simulink library "roller485lib"  (R2023a)
settings: Solver=VariableStepAuto  StartTime=0.0  StopTime=10.0  RelTol=1e-3
libraries: arduinolib x173, simulink x66
(part 2 of 6)

== system roller485lib/I2C Write ==
  note: position mode
  note: current mode
  note: speed mode
  absolute angle command [deg] : Subsystem  mask(absolute angle command [deg]){I2CAddress=0x64, I2CModule=0, position_P=15, position_I=0.000003, position_D=400, set_time1=0, set_time2=0}
      mask prompts: I2CAddress "I2C Address"; I2CModule "I2C Module"; position_P "P"; position_I "I"; position_D "D"; set_time1 "Set Time1"; set_time2 "Set Time2"
      mask help:
      | position mode
      | If t ≤ set_time1, then position mode is set.
      | ---------------------------------
      | default value (PID gain of position controller)
      |  P: 15
      |  I: 0.000003
      |  D: 400
      | If t ≤ set_time2, then PID gain can be set.
      mask TypeOptions I2CModule:
      | Enabled Subsystem
      | (PID setting)/I2C Write
      | (0xA0)/I2CModule | Enabled Subsystem
      | (PID setting)/I2C Write
      | (0xA4)/I2CModule | Enabled Subsystem
      | (PID setting)/I2C Write
      | (0xA8)/I2CModule | Enabled Subsystem
      | (mode setting)/I2C Write
      | (0x01)/I2CModule | I2C Write
      | (0x80)/I2CModule
      mask DialogControl ParameterGroupVar Prompt: パラメーター
      mask Display:
      | image('roller485.png', [55,10,75,56]);
      | 
      | color('blue');
      | text(5, 62, 'absolute position control');
      | text(17, 22, '# mode setting');
      | text(17, 10, '# PID gain setting');
      | color('black');
      | 
      | color('red');
      | addr = get_param(gcb, 'I2CAddress');
      | text(10, 50, ['I2C: ' addr]);
      | 
      | color('red');
      | module = get_param(gcb, 'I2CModule');
      | text(60, 50, ['<I2C' module '>']);
  absolute angle command [deg] and max current [mA] : Subsystem  mask(absolute angle command [deg]){I2CAddress=0x64, I2CModule=0, position_P=15, position_I=0.000003, position_D=400, max_current=1000, set_time1=0, set_time2=0, set_time3=0}
      mask prompts: I2CAddress "I2C Address"; I2CModule "I2C Module"; position_P "P"; position_I "I"; position_D "D"; max_current "Imax [mA]"; set_time1 "Set Time1"; set_time2 "Set Time2"; set_time3 "Set Time3"
      mask help:
      | position mode
      | If t ≤ set_time1, then position mode is set.
      | ---------------------------------
      | default value (PID gain of position controller)
      |  P: 15
      |  I: 0.000003
      |  D: 400
      | If t ≤ set_time2, then PID gain can be set.
      | ---------------------------------
      | default value (Imax: max current)
      |  Imax: 1000 mA
      |   ---> Imax can be set up to a maximum of 1200mA.
      | If t ≤ set_time3, then Imax can be set.
      mask TypeOptions I2CModule:
      | Enabled Subsystem
      | (PID setting)/I2C Write
      | (0xA0)/I2CModule | Enabled Subsystem
      | (PID setting)/I2C Write
      | (0xA4)/I2CModule | Enabled Subsystem
      | (PID setting)/I2C Write
      | (0xA8)/I2CModule | Enabled Subsystem
      | (max current setting)/I2C Write
      | (0x50)/I2CModule | Enabled Subsystem
      | (mode setting)/I2C Write
      | (0x01)/I2CModule | I2C Write
      | (0x80)/I2CModule
      mask DialogControl ParameterGroupVar Prompt: パラメーター
      mask Display:
      | image('roller485.png', [55,10,75,56]);
      | 
      | color('blue');
      | text(5, 62, 'absolute position control');
      | text(17, 22, '# mode setting');
      | text(17, 10, '# PID gain & Imax setting');
      | 
      | color('red');
      | addr = get_param(gcb, 'I2CAddress');
      | text(10, 50, ['I2C: ' addr]);
      | 
      | color('red');
      | module = get_param(gcb, 'I2CModule');
      | text(60, 50, ['<I2C' module '>']);
  absolute angle command [rad] : Subsystem  mask(absolute angle command [rad]){I2CAddress=0x64, I2CModule=0, position_P=15, position_I=0.000003, position_D=400, set_time1=0, set_time2=0}
      mask prompts: I2CAddress "I2C Address"; I2CModule "I2C Module"; position_P "P"; position_I "I"; position_D "D"; set_time1 "Set Time1"; set_time2 "Set Time2"
      mask help:
      | position mode
      | If t ≤ set_time1, then position mode is set.
      | ---------------------------------
      | default value (PID gain of position controller)
      |  P: 15
      |  I: 0.000003
      |  D: 400
      | If t ≤ set_time2, then PID gain can be set.
      mask TypeOptions I2CModule:
      | Enabled Subsystem
      | (PID setting)/I2C Write
      | (0xA0)/I2CModule | Enabled Subsystem
      | (PID setting)/I2C Write
      | (0xA4)/I2CModule | Enabled Subsystem
      | (PID setting)/I2C Write
      | (0xA8)/I2CModule | Enabled Subsystem
      | (mode setting)/I2C Write
      | (0x01)/I2CModule | I2C Write
      | (0x80)/I2CModule
      mask DialogControl ParameterGroupVar Prompt: パラメーター
      mask Display:
      | image('roller485.png', [55,10,75,56]);
      | 
      | color('blue');
      | text(5, 62, 'absolute position control');
      | text(17, 22, '# mode setting');
      | text(17, 10, '# PID gain setting');
      | 
      | color('red');
      | addr = get_param(gcb, 'I2CAddress');
      | text(10, 50, ['I2C: ' addr]);
      | 
      | color('red');
      | module = get_param(gcb, 'I2CModule');
      | text(60, 50, ['<I2C' module '>']);
  absolute angle command [rad] and max current [mA] : Subsystem  mask(absolute angle command [rad]){I2CAddress=0x64, I2CModule=0, position_P=15, position_I=0.000003, position_D=400, max_current=1000, set_time1=0, set_time2=0, set_time3=0}
      mask prompts: I2CAddress "I2C Address"; I2CModule "I2C module:"; position_P "P"; position_I "I"; position_D "D"; max_current "Imax [mA]"; set_time1 "Set Time1"; set_time2 "Set Time2"; set_time3 "Set Time3"
      mask help:
      | position mode
      | If t ≤ set_time1, then position mode is set.
      | ---------------------------------
      | default value (PID gain of position controller)
      |  P: 15
      |  I: 0.000003
      |  D: 400
      | If t ≤ set_time2, then PID gain can be set.
      | ---------------------------------
      | default value (Imax: max current)
      |  Imax: 1000 mA
      |   ---> Imax can be set up to a maximum of 1200mA.
      | If t ≤ set_time3, then Imax can be set.
      mask TypeOptions I2CModule:
      | Enabled Subsystem
      | (PID setting)/I2C Write
      | (0xA0)/I2CModule | Enabled Subsystem
      | (PID setting)/I2C Write
      | (0xA4)/I2CModule | Enabled Subsystem
      | (PID setting)/I2C Write
      | (0xA8)/I2CModule | Enabled Subsystem
      | (max current setting)/I2C Write
      | (0x50)/I2CModule | Enabled Subsystem
      | (mode setting)/I2C Write
      | (0x01)/I2CModule | I2C Write
      | (0x80)/I2CModule
      mask DialogControl ParameterGroupVar Prompt: パラメーター
      mask Display:
      | image('roller485.png', [55,10,75,56]);
      | 
      | color('blue');
      | text(5, 62, 'absolute position control');
      | text(17, 22, '# mode setting');
      | text(17, 10, '# PID gain & Imax setting');
      | 
      | color('red');
      | addr = get_param(gcb, 'I2CAddress');
      | text(10, 50, ['I2C: ' addr]);
      | 
      | color('red');
      | module = get_param(gcb, 'I2CModule');
      | text(60, 50, ['<I2C' module '>']);
  angular velocity command [rad/s] : Subsystem  mask(angular velocity command [rad/s]){I2CAddress=0x64, I2CModule=0, speed_P=15, speed_I=0.0001, speed_D=400, set_time1=0, set_time2=0}
      mask prompts: I2CAddress "I2C Address"; I2CModule "I2C Module"; speed_P "P"; speed_I "I"; speed_D "D"; set_time1 "Set Time1"; set_time2 "Set Time2"
      mask help:
      | speed mode
      | If t ≤ set_time1, then speed mode is set.
      | ---------------------------------
      | default value (PID gain of speed controller)
      |      P: 15,  I: 0.0001,  D: 400
      | recommended value (PID gain of speed controller)
      |      P: 2,  I: 0,  D: 850
      | If t ≤ set_time2, then PID gain can be set.
      mask TypeOptions I2CModule:
      | Enabled Subsystem
      | (PID setting)/I2C Write
      | (0x70)/I2CModule | Enabled Subsystem
      | (PID setting)/I2C Write
      | (0x74)/I2CModule | Enabled Subsystem
      | (PID setting)/I2C Write
      | (0x78)/I2CModule | Enabled Subsystem
      | (mode setting)/I2C Write
      | (0x01)/I2CModule | I2C Write
      | (0x40)/I2CModule
      mask DialogControl ParameterGroupVar Prompt: パラメーター
      mask Display:
      | image('roller485.png', [55,10,75,56]);
      | 
      | color('green');
      | text(5, 62, 'speed control');
      | text(17, 22, '# mode setting');
      | text(17, 10, '# PID gain setting');
      | 
      | color('red');
      | addr = get_param(gcb, 'I2CAddress');
      | text(10, 50, ['I2C: ' addr]);
      | 
      | color('red');
      | module = get_param(gcb, 'I2CModule');
      | text(60, 50, ['<I2C' module '>']);
  angular velocity command [rad/s] and max current [mA] : Subsystem  mask(angular velocity command [rad/s]){I2CAddress=0x64, I2CModule=0, speed_P=15, speed_I=0.0001, speed_D=400, max_current=1000, set_time1=0, set_time2=0, set_time3=0}
      mask prompts: I2CAddress "I2C Address"; I2CModule "I2C Module"; speed_P "P"; speed_I "I"; speed_D "D"; max_current "Imax [mA]"; set_time1 "Set Time1"; set_time2 "Set Time2"; set_time3 "Set Time3"
      mask help:
      | speed mode
      | If t ≤ set_time1, then speed mode is set.
      | ---------------------------------
      | default value (PID gain of speed controller)
      |      P: 15,  I: 0.0001,  D: 400
      | recommended value (PID gain of speed controller)
      |      P: 2,  I: 0,  D: 850
      | If t ≤ set_time2, then PID gain and Imax can be set.
      | ---------------------------------
      | default value (Imax: max current)
      |  Imax: 1000 mA
      |  ---> Imax can be set up to a maximum of 1200mA.
      | If t ≤ set_time3, then Imax is set.
      mask TypeOptions I2CModule:
      | Enabled Subsystem
      | (PID setting)/I2C Write
      | (0x70)/I2CModule | Enabled Subsystem
      | (PID setting)/I2C Write
      | (0x74)/I2CModule | Enabled Subsystem
      | (PID setting)/I2C Write
      | (0x78)/I2CModule | Enabled Subsystem
      | (max current setting)/I2C Write
      | (0x50)/I2CModule | Enabled Subsystem
      | (mode setting)/I2C Write
      | (0x01)/I2CModule | I2C Write
      | (0x40)/I2CModule
      mask DialogControl ParameterGroupVar Prompt: パラメーター
      mask Display:
      | image('roller485.png', [55,10,75,56]);
      | 
      | color('green');
      | text(5, 62, 'speed control');
      | text(17, 22, '# mode setting');
      | text(17, 10, '# PID gain & Imax setting');
      | 
      | color('red');
      | addr = get_param(gcb, 'I2CAddress');
      | text(10, 50, ['I2C: ' addr]);
      | 
      | color('red');
      | module = get_param(gcb, 'I2CModule');
      | text(60, 50, ['<I2C' module '>']);
  angular velocity command [rpm] : Subsystem  mask(angular velocity command [rad/s]){I2CAddress=0x64, I2CModule=0, speed_P=15, speed_I=0.0001, speed_D=400, set_time1=0, set_time2=0}
      mask prompts: I2CAddress "I2C Address"; I2CModule "I2C Module"; speed_P "P"; speed_I "I"; speed_D "D"; set_time1 "Set Time1"; set_time2 "Set Time2"
      mask help:
      | speed mode
      | If t ≤ set_time1, then speed mode is set.
      | ---------------------------------
      | default value (PID gain of speed controller)
      |      P: 15,  I: 0.0001,  D: 400
      | recommended value (PID gain of speed controller)
      |      P: 2,  I: 0,  D: 850
      | If t ≤ set_time2, then PID gain can be set.
      mask TypeOptions I2CModule:
      | Enabled Subsystem
      | (PID setting)/I2C Write
      | (0x70)/I2CModule | Enabled Subsystem
      | (PID setting)/I2C Write
      | (0x74)/I2CModule | Enabled Subsystem
      | (PID setting)/I2C Write
      | (0x78)/I2CModule | Enabled Subsystem
      | (mode setting)/I2C Write
      | (0x01)/I2CModule | I2C Write
      | (0x40)/I2CModule
      mask DialogControl ParameterGroupVar Prompt: パラメーター
      mask Display:
      | image('roller485.png', [55,10,75,56]);
      | 
      | color('green');
      | text(5, 62, 'speed control');
      | text(17, 22, '# mode setting');
      | text(17, 10, '# PID gain setting');
      | 
      | color('red');
      | addr = get_param(gcb, 'I2CAddress');
      | text(10, 50, ['I2C: ' addr]);
      | 
      | color('red');
      | module = get_param(gcb, 'I2CModule');
      | text(60, 50, ['<I2C' module '>']);
  angular velocity command [rpm] and max current [mA] : Subsystem  mask(angular velocity command [rpm]){I2CAddress=0x64, I2CModule=0, speed_P=15, speed_I=0.0001, speed_D=400, max_current=1000, set_time1=0, set_time2=0, set_time3=0}
      mask prompts: I2CAddress "I2C Address"; I2CModule "I2C Module"; speed_P "P"; speed_I "I"; speed_D "D"; max_current "Imax [mA]"; set_time1 "Set Time1"; set_time2 "Set Time2"; set_time3 "Set Time3"
      mask help:
      | speed mode
      | If t ≤ set_time1, then speed mode is set.
      | ---------------------------------
      | default value (PID gain of speed controller)
      |      P: 15,  I: 0.0001,  D: 400
      | recommended value (PID gain of speed controller)
      |      P: 2,  I: 0,  D: 850
      | If t ≤ set_time2, then PID gain and Imax can be set.
      | ---------------------------------
      | default value (Imax: max current)
      |  Imax: 1000 mA
      |  ---> Imax can be set up to a maximum of 1200mA.
      | If t ≤ set_time3, then Imax is set.
      mask TypeOptions I2CModule:
      | Enabled Subsystem
      | (PID setting)/I2C Write
      | (0x70)/I2CModule | Enabled Subsystem
      | (PID setting)/I2C Write
      | (0x74)/I2CModule | Enabled Subsystem
      | (PID setting)/I2C Write
      | (0x78)/I2CModule | Enabled Subsystem
      | (max current setting)/I2C Write
      | (0x50)/I2CModule | Enabled Subsystem
      | (mode setting)/I2C Write
      | (0x01)/I2CModule | I2C Write
      | (0x40)/I2CModule
      mask DialogControl ParameterGroupVar Prompt: パラメーター
      mask Display:
      | image('roller485.png', [55,10,75,56]);
      | color('green');
      | text(5, 62, 'speed control');
      | 
      | text(17, 22, '# mode setting');
      | text(17, 10, '# PID gain & Imax setting');
      | 
      | color('red');
      | addr = get_param(gcb, 'I2CAddress');
      | text(10, 50, ['I2C: ' addr]);
      | 
      | color('red');
      | module = get_param(gcb, 'I2CModule');
      | text(60, 50, ['<I2C' module '>']);
  current command [A] : Subsystem  mask(current command [A]){I2CAddress=0x64, I2CModule=0, set_time=0}
      mask prompts: I2CAddress "I2C Address"; I2CModule "I2C Module"; set_time "Set Time"
      mask help:
      | current mode
      | If t ≤ set_time, then current mode is set.
      | ---------------------------------
      | PID gain of current controller
      |  P: 0.002
      |  I: 0.00005
      |  D: 0
      | Changing the PID gains is not permitted.
      mask TypeOptions I2CModule:
      | Enabled Subsystem
      | (mode setting)/I2C Write
      | (0x01)/I2CModule | I2C Write
      | (0xB0)/I2CModule
      mask DialogControl ParameterGroupVar Prompt: パラメーター
      mask Display:
      | image('roller485.png', [55,10,75,56]);
      | 
      | color('orange');
      | text(5, 62, 'current control');
      | text(17, 22, '# mode setting');
      | 
      | color('red');
      | addr = get_param(gcb, 'I2CAddress');
      | text(10, 50, ['I2C: ' addr]);
      | 
      | color('red');
      | module = get_param(gcb, 'I2CModule');
      | text(60, 50, ['<I2C' module '>']);
  current command [mA] : Subsystem  mask(current command [A]){I2CAddress=0x64, I2CModule=0, set_time=0}
      mask prompts: I2CAddress "I2C Address"; I2CModule "I2C Module"; set_time "Set Time"
      mask help:
      | current mode
      | If t ≤ set_time, then current mode is set.
      | ---------------------------------
      | PID gain of current controller
      |  P: 0.002
      |  I: 0.00005
      |  D: 0
      | Changing the PID gains is not permitted.
      mask TypeOptions I2CModule:
      | Enabled Subsystem
      | (mode setting)/I2C Write
      | (0x01)/I2CModule | I2C Write
      | (0xB0)/I2CModule
      mask DialogControl ParameterGroupVar Prompt: パラメーター
      mask Display:
      | image('roller485.png', [55,10,75,56]);
      | 
      | color('orange');
      | text(5, 62, 'current control');
      | text(17, 22, '# mode setting');
      | 
      | color('red');
      | addr = get_param(gcb, 'I2CAddress');
      | text(10, 50, ['I2C: ' addr]);
      | 
      | color('red');
      | module = get_param(gcb, 'I2CModule');
      | text(60, 50, ['<I2C' module '>']);
  relative angle command [deg] : Subsystem  mask(relative angle command [deg]){I2CAddress=0x64, I2CModule=0, sample_time=-1, position_P=15, position_I=0.000003, position_D=400, set_time1=0, set_time2=0}
      mask prompts: I2CAddress "I2C Address"; I2CModule "I2C Module"; sample_time "Sample Time (-1 for inherited)"; position_P "P"; position_I "I"; position_D "D"; set_time1 "Set Time1"; set_time2 "Set Time2"
      mask help:
      | position mode
      | If t ≤ set_time1, then position mode and initial angle are set.
      | ---------------------------------
      | default value (PID gain of position controller)
      |  P: 15
      |  I: 0.000003
      |  D: 400
      | If t ≤ set_time2, then PID gain can be set.
      mask TypeOptions I2CModule:
      | Enabled Subsystem
      | (PID setting)/I2C Write
      | (0xA0)/I2CModule | Enabled Subsystem
      | (PID setting)/I2C Write
      | (0xA4)/I2CModule | Enabled Subsystem
      | (PID setting)/I2C Write
      | (0xA8)/I2CModule | Enabled Subsystem
      | (initialization angle)/I2C Read
      | (0x90)/I2CModule | Enabled Subsystem
      | (mode setting)/I2C Write
      | (0x01)/I2CModule | I2C Write
      | (0x80)/I2CModule
      mask DialogControl ParameterGroupVar Prompt: パラメーター
      mask Display:
      | image('roller485.png', [55,10,75,56]);
      | 
      | color('blue');
      | text(5, 62, 'relative position control');
      | text(17, 22, '# mode setting');
      | text(17, 10, '# PID gain setting');
      | 
      | color('red');
      | addr = get_param(gcb, 'I2CAddress');
      | text(10, 50, ['I2C: ' addr]);
      | 
      | color('red');
      | module = get_param(gcb, 'I2CModule');
      | text(60, 50, ['<I2C' module '>']);
  relative angle command [deg] and max current [mA] : Subsystem  mask(relative angle command [rad]){I2CAddress=0x64, I2CModule=0, sample_time=-1, position_P=15, position_I=0.000003, position_D=400, max_current=1000, set_time1=0, set_time2=0, set_time3=0}
      mask prompts: I2CAddress "I2C Address"; I2CModule "I2C module:"; sample_time "Sample Time (-1 for inherited)"; position_P "P"; position_I "I"; position_D "D"; max_current "Imax [mA]"; set_time1 "Set Time1"; set_time2 "Set Time2"; set_time3 "Set Time3"
      mask help:
      | position mode
      | If t ≤ set_time1, then position mode and initial angle are set.
      | ---------------------------------
      | default value (PID gain of position controller)
      |  P: 15
      |  I: 0.000003
      |  D: 400
      | If t ≤ set_time2, then PID gain can be set.
      | ---------------------------------
      | default value (Imax: max current)
      |  Imax: 1000 mA
      |   ---> Imax can be set up to a maximum of 1200mA.
      | If t ≤ set_time3, then Imax can be set.
      mask TypeOptions I2CModule:
      | Enabled Subsystem
      | (PID setting)/I2C Write
      | (0xA0)/I2CModule | Enabled Subsystem
      | (PID setting)/I2C Write
      | (0xA4)/I2CModule | Enabled Subsystem
      | (PID setting)/I2C Write
      | (0xA8)/I2CModule | Enabled Subsystem
      | (initialization angle)/I2C Read
      | (0x90)/I2CModule | Enabled Subsystem
      | (max current setting)/I2C Write
      | (0x50)/I2CModule | Enabled Subsystem
      | (mode setting)/I2C Write
      | (0x01)/I2CModule | I2C Write
      | (0x80)/I2CModule
      mask DialogControl ParameterGroupVar Prompt: パラメーター
      mask Display:
      | image('roller485.png', [55,10,75,56]);
      | 
      | color('blue');
      | text(5, 62, 'relative position control');
      | text(17, 22, '# mode setting');
      | text(17, 10, '# PID gain & Imax setting');
      | 
      | color('red');
      | addr = get_param(gcb, 'I2CAddress');
      | text(10, 50, ['I2C: ' addr]);
      | 
      | color('red');
      | module = get_param(gcb, 'I2CModule');
      | text(60, 50, ['<I2C' module '>']);
  relative angle command [rad] : Subsystem  mask(relative angle command [rad]){I2CAddress=0x64, I2CModule=0, sample_time=-1, position_P=15, position_I=0.000003, position_D=400, set_time1=0, set_time2=0}
      mask prompts: I2CAddress "I2C Address"; I2CModule "I2C Module"; sample_time "Sample Time (-1 for inherited)"; position_P "P"; position_I "I"; position_D "D"; set_time1 "Set Time1"; set_time2 "Set Time2"
      mask help:
      | position mode
      | If t ≤ set_time1, then position mode and initial angle are set.
      | ---------------------------------
      | default value (PID gain of position controller)
      |  P: 15
      |  I: 0.000003
      |  D: 400
      | If t ≤ set_time2, then PID gain can be set.
      mask TypeOptions I2CModule:
      | Enabled Subsystem
      | (PID setting)/I2C Write
      | (0xA0)/I2CModule | Enabled Subsystem
      | (PID setting)/I2C Write
      | (0xA4)/I2CModule | Enabled Subsystem
      | (PID setting)/I2C Write
      | (0xA8)/I2CModule | Enabled Subsystem
      | (initialization angle)/I2C Read
      | (0x90)/I2CModule | Enabled Subsystem
      | (mode setting)/I2C Write
      | (0x01)/I2CModule | I2C Write
      | (0x80)/I2CModule
      mask DialogControl ParameterGroupVar Prompt: パラメーター
      mask Display:
      | image('roller485.png', [55,10,75,56]);
      | 
      | color('blue');
      | text(5, 62, 'relative position control');
      | text(17, 22, '# mode setting');
      | text(17, 10, '# PID gain setting');
      | 
      | color('red');
      | addr = get_param(gcb, 'I2CAddress');
      | text(10, 50, ['I2C: ' addr]);
      | 
      | color('red');
      | module = get_param(gcb, 'I2CModule');
      | text(60, 50, ['<I2C' module '>']);
  relative angle command [rad] and max current [mA] : Subsystem  mask(relative angle command [rad]){I2CAddress=0x64, I2CModule=0, sample_time=-1, position_P=15, position_I=0.000003, position_D=400, max_current=1000, set_time1=0, set_time2=0, set_time3=0}
      mask prompts: I2CAddress "I2C Address"; I2CModule "I2C Module"; sample_time "Sample Time (-1 for inherited)"; position_P "P"; position_I "I"; position_D "D"; max_current "Imax [mA]"; set_time1 "Set Time1"; set_time2 "Set Time2"; set_time3 "Set Time3"
      mask help:
      | position mode
      | If t ≤ set_time1, then position mode and initial angle are set.
      | ---------------------------------
      | default value (PID gain of position controller)
      |  P: 15
      |  I: 0.000003
      |  D: 400
      | If t ≤ set_time2, then PID gain can be set.
      | ---------------------------------
      | default value (Imax: max current)
      |  Imax: 1000 mA
      |   ---> Imax can be set up to a maximum of 1200mA.
      | If t ≤ set_time3, then Imax can be set.
      mask TypeOptions I2CModule:
      | Enabled Subsystem
      | (PID setting)/I2C Write
      | (0xA0)/I2CModule | Enabled Subsystem
      | (PID setting)/I2C Write
      | (0xA4)/I2CModule | Enabled Subsystem
      | (PID setting)/I2C Write
      | (0xA8)/I2CModule | Enabled Subsystem
      | (initialization angle)/I2C Read
      | (0x90)/I2CModule | Enabled Subsystem
      | (max current setting)/I2C Write
      | (0x50)/I2CModule | Enabled Subsystem
      | (mode setting)/I2C Write
      | (0x01)/I2CModule | I2C Write
      | (0x80)/I2CModule
      mask DialogControl ParameterGroupVar Prompt: パラメーター
      mask Display:
      | image('roller485.png', [55,10,75,56]);
      | 
      | color('blue');
      | text(5, 62, 'relative position control');
      | text(17, 22, '# mode setting');
      | text(17, 10, '# PID gain & Imax setting');
      | 
      | color('red');
      | addr = get_param(gcb, 'I2CAddress');
      | text(10, 50, ['I2C: ' addr]);
      | 
      | color('red');
      | module = get_param(gcb, 'I2CModule');
      | text(60, 50, ['<I2C' module '>']);

== system roller485lib/I2C Write (using MATLAB Function) ==
  note: speed mode
  note: current mode
  note: position mode
  absolute angle command [deg] (using MATLAB Function) : Subsystem  mask(absolute angle command [deg]){I2CAddress=0x64, I2CModule=0, position_P=15, position_I=0.000003, position_D=400, set_time1=0, set_time2=0}
      mask prompts: I2CAddress "I2C Address"; I2CModule "I2C Module"; position_P "P"; position_I "I"; position_D "D"; set_time1 "Set Time1"; set_time2 "Set Time2"
      mask help:
      | position mode
      | If t ≤ set_time1, then position mode is set.
      | ---------------------------------
      | default value (PID gain of position controller)
      |  P: 15
      |  I: 0.000003
      |  D: 400
      | If t ≤ set_time2, then PID gain can be set.
      mask TypeOptions I2CModule:
      | Enabled Subsystem
      | (PID setting)/I2C Write
      | (0xA0)/I2CModule | Enabled Subsystem
      | (PID setting)/I2C Write
      | (0xA4)/I2CModule | Enabled Subsystem
      | (PID setting)/I2C Write
      | (0xA8)/I2CModule | Enabled Subsystem
      | (mode setting)/I2C Write
      | (0x01)/I2CModule | I2C Write
      | (0x80)/I2CModule
      mask DialogControl ParameterGroupVar Prompt: パラメーター
      mask Display:
      | image('roller485_matlab_fcn2.png', [55,10,75,56]);
      | 
      | color('blue');
      | text(5, 62, 'absolute position control');
      | text(17, 22, '# mode setting');
      | text(17, 10, '# PID gain setting');
      | 
      | color('red');
      | addr = get_param(gcb, 'I2CAddress');
      | text(10, 50, ['I2C: ' addr]);
      | 
      | color('red');
      | module = get_param(gcb, 'I2CModule');
      | text(60, 50, ['<I2C' module '>']);
  absolute angle command [rad] (using MATLAB Function) : Subsystem  mask(absolute angle command [rad]){I2CAddress=0x64, I2CModule=0, position_P=15, position_I=0.000003, position_D=400, set_time1=0, set_time2=0}
      mask prompts: I2CAddress "I2C Address"; I2CModule "I2C Module"; position_P "P"; position_I "I"; position_D "D"; set_time1 "Set Time1"; set_time2 "Set Time2"
      mask help:
      | position mode
      | If t ≤ set_time1, then position mode is set.
      | ---------------------------------
      | default value (PID gain of position controller)
      |  P: 15
      |  I: 0.000003
      |  D: 400
      | If t ≤ set_time2, then PID gain can be set.
      mask TypeOptions I2CModule:
      | Enabled Subsystem
      | (PID setting)/I2C Write
      | (0xA0)/I2CModule | Enabled Subsystem
      | (PID setting)/I2C Write
      | (0xA4)/I2CModule | Enabled Subsystem
      | (PID setting)/I2C Write
      | (0xA8)/I2CModule | Enabled Subsystem
      | (mode setting)/I2C Write
      | (0x01)/I2CModule | I2C Write
      | (0x80)/I2CModule
      mask DialogControl ParameterGroupVar Prompt: パラメーター
      mask Display:
      | image('roller485_matlab_fcn2.png', [55,10,75,56]);
      | 
      | color('blue');
      | text(5, 62, 'absolute position control');
      | text(17, 22, '# mode setting');
      | text(17, 10, '# PID gain setting');
      | 
      | color('red');
      | addr = get_param(gcb, 'I2CAddress');
      | text(10, 50, ['I2C: ' addr]);
      | 
      | color('red');
      | module = get_param(gcb, 'I2CModule');
      | text(60, 50, ['<I2C' module '>']);
  angular velocity command [rad/s] (using MATLAB Function) : Subsystem  mask(angular velocity command [rad/s]){I2CAddress=0x64, I2CModule=0, speed_P=15, speed_I=0.0001, speed_D=400, set_time1=0, set_time2=0}
      mask prompts: I2CAddress "I2C Address"; I2CModule "I2C Module"; speed_P "P"; speed_I "I"; speed_D "D"; set_time1 "Set Time1"; set_time2 "Set Time2"
      mask help:
      | speed mode
      | If t ≤ set_time1, then speed mode is set.
      | ---------------------------------
      | default value (PID gain of speed controller)
      |      P: 15,  I: 0.0001,  D: 400
      | recommended value (PID gain of speed controller)
      |      P: 2,  I: 0,  D: 850
      | If t ≤ set_time2, then PID gain can be set.
      mask TypeOptions I2CModule:
      | Enabled Subsystem
      | (PID setting)/I2C Write
      | (0x70)/I2CModule | Enabled Subsystem
      | (PID setting)/I2C Write
      | (0x74)/I2CModule | Enabled Subsystem
      | (PID setting)/I2C Write
      | (0x78)/I2CModule | Enabled Subsystem
      | (mode setting)/I2C Write
      | (0x01)/I2CModule | I2C Write
      | (0x40)/I2CModule
      mask DialogControl ParameterGroupVar Prompt: パラメーター
      mask Display:
      | image('roller485_matlab_fcn2.png', [55,10,75,56]);
      | 
      | color('green');
      | text(5, 62, 'speed control');
      | text(17, 22, '# mode setting');
      | text(17, 10, '# PID gain setting');
      | 
      | color('red');
      | addr = get_param(gcb, 'I2CAddress');
      | text(10, 50, ['I2C: ' addr]);
      | 
      | color('red');
      | module = get_param(gcb, 'I2CModule');
      | text(60, 50, ['<I2C' module '>']);
  angular velocity command [rpm] (using MATLAB Function) : Subsystem  mask(angular velocity command [rpm]){I2CAddress=0x64, I2CModule=0, speed_P=15, speed_I=0.0001, speed_D=400, set_time1=0, set_time2=0}
      mask prompts: I2CAddress "I2C Address"; I2CModule "I2C Module"; speed_P "P"; speed_I "I"; speed_D "D"; set_time1 "Set Time1"; set_time2 "Set Time2"
      mask help:
      | speed mode
      | If t ≤ set_time1, then speed mode is set.
      | ---------------------------------
      | default value (PID gain of speed controller)
      |      P: 15,  I: 0.0001,  D: 400
      | recommended value (PID gain of speed controller)
      |      P: 2,  I: 0,  D: 850
      | If t ≤ set_time2, then PID gain can be set.
      mask TypeOptions I2CModule:
      | Enabled Subsystem
      | (PID setting)/I2C Write
      | (0x70)/I2CModule | Enabled Subsystem
      | (PID setting)/I2C Write
      | (0x74)/I2CModule | Enabled Subsystem
      | (PID setting)/I2C Write
      | (0x78)/I2CModule | Enabled Subsystem
      | (mode setting)/I2C Write
      | (0x01)/I2CModule | I2C Write
      | (0x40)/I2CModule
      mask DialogControl ParameterGroupVar Prompt: パラメーター
      mask Display:
      | image('roller485_matlab_fcn2.png', [55,10,75,56]);
      | 
      | color('green');
      | text(5, 62, 'speed control');
      | text(17, 22, '# mode setting');
      | text(17, 10, '# PID gain setting');
      | 
      | color('red');
      | addr = get_param(gcb, 'I2CAddress');
      | text(10, 50, ['I2C: ' addr]);
      | 
      | color('red');
      | module = get_param(gcb, 'I2CModule');
      | text(60, 50, ['<I2C' module '>']);
  current command [A] (using MATLAB Function) : Subsystem  mask(current command [A]){I2CAddress=0x64, I2CModule=0, set_time=0}
      mask prompts: I2CAddress "I2C Address"; I2CModule "I2C Module"; set_time "Set Time"
      mask help:
      | current mode
      | If t ≤ set_time, then current mode is set.
      | ---------------------------------
      | PID gain of current controller
      |  P: 0.002
      |  I: 0.00005
      |  D: 0
      | Changing the PID gains is not permitted.
      mask TypeOptions I2CModule:
      | Enabled Subsystem
      | (mode setting)/I2C Write
      | (0x01)/I2CModule | I2C Write
      | (0xB0)/I2CModule
      mask DialogControl ParameterGroupVar Prompt: パラメーター
      mask Display:
      | image('roller485_matlab_fcn2.png', [55,10,75,56]);
      | 
      | color('orange');
      | text(5, 62, 'current control');
      | text(17, 22, '# mode setting');
      | 
      | color('red');
      | addr = get_param(gcb, 'I2CAddress');
      | text(10, 50, ['I2C: ' addr]);
      | 
      | color('red');
      | module = get_param(gcb, 'I2CModule');
      | text(60, 50, ['<I2C' module '>']);
  current command [mA] (using MATLAB Function) : Subsystem  mask(current command [A]){I2CAddress=0x64, I2CModule=0, set_time=0}
      mask prompts: I2CAddress "I2C Address"; I2CModule "I2C Module"; set_time "Set Time"
      mask help:
      | current mode
      | If t ≤ set_time, then current mode is set.
      | ---------------------------------
      | PID gain of current controller
      |  P: 0.002
      |  I: 0.00005
      |  D: 0
      | Changing the PID gains is not permitted.
      mask TypeOptions I2CModule:
      | Enabled Subsystem
      | (mode setting)/I2C Write
      | (0x01)/I2CModule | I2C Write
      | (0xB0)/I2CModule
      mask DialogControl ParameterGroupVar Prompt: パラメーター
      mask Display:
      | image('roller485_matlab_fcn2.png', [55,10,75,56]);
      | 
      | color('orange');
      | text(5, 62, 'current control');
      | text(17, 22, '# mode setting');
      | 
      | color('red');
      | addr = get_param(gcb, 'I2CAddress');
      | text(10, 50, ['I2C: ' addr]);
      | 
      | color('red');
      | module = get_param(gcb, 'I2CModule');
      | text(60, 50, ['<I2C' module '>']);
  relative angle command [deg] (using MATLAB Function) : Subsystem  mask(relative angle command [deg]){I2CAddress=0x64, I2CModule=0, sample_time=-1, position_P=15, position_I=0.000003, position_D=400, set_time1=0, set_time2=0}
      mask prompts: I2CAddress "I2C Address"; I2CModule "I2C Module"; sample_time "Sample Time (-1 for inherited)"; position_P "P"; position_I "I"; position_D "D"; set_time1 "Set Time1"; set_time2 "Set Time2"
      mask help:
      | position mode
      | If t ≤ set_time1, then position mode and initial angle are set.
      | ---------------------------------
      | default value (PID gain of position controller)
      |  P: 15
      |  I: 0.000003
      |  D: 400
      | If t ≤ set_time2, then PID gain can be set.
      mask TypeOptions I2CModule:
      | Enabled Subsystem
      | (PID setting)/I2C Write
      | (0xA0)/I2CModule | Enabled Subsystem
      | (PID setting)/I2C Write
      | (0xA4)/I2CModule | Enabled Subsystem
      | (PID setting)/I2C Write
      | (0xA8)/I2CModule | Enabled Subsystem
      | (initialization angle)/I2C Read
      | (0x90)/I2CModule | Enabled Subsystem
      | (mode setting)/I2C Write
      | (0x01)/I2CModule | I2C Write
      | (0x80)/I2CModule
      mask DialogControl ParameterGroupVar Prompt: パラメーター
      mask Display:
      | image('roller485_matlab_fcn2.png', [55,10,75,56]);
      | 
      | color('blue');
      | text(5, 62, 'relative position control');
      | text(17, 22, '# mode setting');
      | text(17, 10, '# PID gain setting');
      | 
      | color('red');
      | addr = get_param(gcb, 'I2CAddress');
      | text(10, 50, ['I2C: ' addr]);
      | 
      | color('red');
      | module = get_param(gcb, 'I2CModule');
      | text(60, 50, ['<I2C' module '>']);
  relative angle command [rad] (using MATLAB Function) : Subsystem  mask(relative angle command [rad]){I2CAddress=0x64, I2CModule=0, sample_time=-1, position_P=15, position_I=0.000003, position_D=400, set_time1=0, set_time2=0}
      mask prompts: I2CAddress "I2C Address"; I2CModule "I2C Module"; sample_time "Sample Time (-1 for inherited)"; position_P "P"; position_I "I"; position_D "D"; set_time1 "Set Time1"; set_time2 "Set Time2"
      mask help:
      | position mode
      | If t ≤ set_time1, then position mode and initial angle are set.
      | ---------------------------------
      | default value (PID gain of position controller)
      |  P: 15
      |  I: 0.000003
      |  D: 400
      | If t ≤ set_time2, then PID gain can be set.
      mask TypeOptions I2CModule:
      | Enabled Subsystem
      | (PID setting)/I2C Write
      | (0xA0)/I2CModule | Enabled Subsystem
      | (PID setting)/I2C Write
      | (0xA4)/I2CModule | Enabled Subsystem
      | (PID setting)/I2C Write
      | (0xA8)/I2CModule | Enabled Subsystem
      | (initialization angle)/I2C Read
      | (0x90)/I2CModule | Enabled Subsystem
      | (mode setting)/I2C Write
      | (0x01)/I2CModule | I2C Write
      | (0x80)/I2CModule
      mask DialogControl ParameterGroupVar Prompt: パラメーター
      mask Display:
      | image('roller485_matlab_fcn2.png', [55,10,75,56]);
      | 
      | color('blue');
      | text(5, 62, 'relative position control');
      | text(17, 22, '# mode setting');
      | text(17, 10, '# PID gain setting');
      | 
      | color('red');
      | addr = get_param(gcb, 'I2CAddress');
      | text(10, 50, ['I2C: ' addr]);
      | 
      | color('red');
      | module = get_param(gcb, 'I2CModule');
      | text(60, 50, ['<I2C' module '>']);

== system roller485lib/control mode ==
  Data Type Conversion : DataTypeConversion  OutDataTypeStr=uint8  SaturateOnIntegerOverflow=off  RndMeth=Floor
  I2C Write (0x01) : arduinolib/I2C Write  I2CModule=0  Mode=Master  SlaveAddress=I2CAddress  SlaveByteOrder=BigEndian  Direction=Transmitter  RegisterAddressMode=on  RegisterAddress=0x01  SlaveDataType=uint8  DataLength=1  NoAck=off  RepeatedStart=off  OutputStatus=off  blockPlatform=ARDUINO
  mode : Constant  Value=control_mode
  wires:
  Data Type Conversion/1 -> I2C Write (0x01)/1
  mode/1 -> Data Type Conversion/1

== system roller485lib/control mode (initial time only) ==
  Clock : Clock
  Compare To Constant : simulink/Logic and Bit Operations/Compare To Constant  relop===  const=0  OutDataTypeStr=boolean
  Enabled Subsystem : Subsystem  TreatAsAtomicUnit=on
  mode : Constant  Value=control_mode
  wires:
  mode/1 -> Enabled Subsystem/1(mode)
  Compare To Constant/1 -> Enabled Subsystem/Enable
  Clock/1 -> Compare To Constant/1

== system roller485lib/motor ON//OFF ==
  ON (1) or OFF (0) : Inport
  Data Type Conversion : DataTypeConversion  OutDataTypeStr=uint8  SaturateOnIntegerOverflow=off  RndMeth=Floor
  I2C Write (0x00) : arduinolib/I2C Write  I2CModule=0  Mode=Master  SlaveAddress=I2CAddress  SlaveByteOrder=BigEndian  Direction=Transmitter  RegisterAddressMode=on  RegisterAddress=0x00  SlaveDataType=uint8  DataLength=1  NoAck=off  RepeatedStart=off  OutputStatus=off  blockPlatform=ARDUINO
  wires:
  Data Type Conversion/1 -> I2C Write (0x00)/1
  ON (1) or OFF (0)/1 -> Data Type Conversion/1

== system roller485lib/Basic I2C Write/basic absolute angle command [deg] ==
  command [deg] : Inport
  Data Type Conversion : DataTypeConversion  OutDataTypeStr=uint32  SaturateOnIntegerOverflow=off  RndMeth=Floor
  I2C Write (0x80) : arduinolib/I2C Write  I2CModule=0  Mode=Master  SlaveAddress=I2CAddress  SlaveByteOrder=LittleEndian  Direction=Transmitter  RegisterAddressMode=on  RegisterAddress=0x80  SlaveDataType=uint8  DataLength=1  NoAck=off  RepeatedStart=off  OutputStatus=off  blockPlatform=ARDUINO
  x 100 : Gain  Gain=100
  wires:
  command [deg]/1 -> x 100/1
  Data Type Conversion/1 -> I2C Write (0x80)/1
  x 100/1 -> Data Type Conversion/1

== system roller485lib/Basic I2C Write/basic absolute angle command [rad] ==
  command [rad] : Inport
  Data Type Conversion : DataTypeConversion  OutDataTypeStr=uint32  SaturateOnIntegerOverflow=off  RndMeth=Floor
  I2C Write (0x80) : arduinolib/I2C Write  I2CModule=0  Mode=Master  SlaveAddress=I2CAddress  SlaveByteOrder=LittleEndian  Direction=Transmitter  RegisterAddressMode=on  RegisterAddress=0x80  SlaveDataType=uint8  DataLength=1  NoAck=off  RepeatedStart=off  OutputStatus=off  blockPlatform=ARDUINO
  rad to deg : Gain  Gain=180/pi
  x 100 : Gain  Gain=100
  wires:
  command [rad]/1 -> rad to deg/1
  rad to deg/1 -> x 100/1
  Data Type Conversion/1 -> I2C Write (0x80)/1
  x 100/1 -> Data Type Conversion/1

== system roller485lib/Basic I2C Write/basic angular velocity command [rad//s] ==
  command [rad/s] : Inport
  Data Type Conversion2 : DataTypeConversion  OutDataTypeStr=uint32  SaturateOnIntegerOverflow=off  RndMeth=Floor
  I2C Write (0x40) : arduinolib/I2C Write  I2CModule=0  Mode=Master  SlaveAddress=I2CAddress  SlaveByteOrder=LittleEndian  Direction=Transmitter  RegisterAddressMode=on  RegisterAddress=0x40  SlaveDataType=uint8  DataLength=1  NoAck=off  RepeatedStart=off  OutputStatus=off  blockPlatform=ARDUINO
  rad/s to rpm : Gain  Gain=60/(2*pi)
  x 100 : Gain  Gain=100
  wires:
  command [rad/s]/1 -> rad/s to rpm/1
  rad/s to rpm/1 -> x 100/1
  Data Type Conversion2/1 -> I2C Write (0x40)/1
  x 100/1 -> Data Type Conversion2/1

== system roller485lib/Basic I2C Write/basic angular velocity command [rpm] ==
  command [rpm] : Inport
  Data Type Conversion : DataTypeConversion  OutDataTypeStr=uint32  SaturateOnIntegerOverflow=off  RndMeth=Floor
  I2C Write (0x40) : arduinolib/I2C Write  I2CModule=0  Mode=Master  SlaveAddress=I2CAddress  SlaveByteOrder=LittleEndian  Direction=Transmitter  RegisterAddressMode=on  RegisterAddress=0x40  SlaveDataType=uint8  DataLength=1  NoAck=off  RepeatedStart=off  OutputStatus=off  blockPlatform=ARDUINO
  x 100 : Gain  Gain=100
  wires:
  x 100/1 -> Data Type Conversion/1
  command [rpm]/1 -> x 100/1
  Data Type Conversion/1 -> I2C Write (0x40)/1

== system roller485lib/Basic I2C Write/basic current command [A] ==
  command [A] : Inport
  A to mA : Gain  Gain=1000
  Data Type Conversion : DataTypeConversion  OutDataTypeStr=uint32  SaturateOnIntegerOverflow=off  RndMeth=Floor
  I2C Write (0xB0) : arduinolib/I2C Write  I2CModule=0  Mode=Master  SlaveAddress=I2CAddress  SlaveByteOrder=LittleEndian  Direction=Transmitter  RegisterAddressMode=on  RegisterAddress=0xB0  SlaveDataType=uint8  DataLength=1  NoAck=off  RepeatedStart=off  OutputStatus=off  blockPlatform=ARDUINO
  x 100 : Gain  Gain=100
  wires:
  command [A]/1 -> A to mA/1
  A to mA/1 -> x 100/1
  Data Type Conversion/1 -> I2C Write (0xB0)/1
  x 100/1 -> Data Type Conversion/1

== system roller485lib/Basic I2C Write/basic current command [mA] ==
  command [mA] : Inport
  Data Type Conversion : DataTypeConversion  OutDataTypeStr=uint32  SaturateOnIntegerOverflow=off  RndMeth=Floor
  I2C Write (0xB0) : arduinolib/I2C Write  I2CModule=0  Mode=Master  SlaveAddress=I2CAddress  SlaveByteOrder=LittleEndian  Direction=Transmitter  RegisterAddressMode=on  RegisterAddress=0xB0  SlaveDataType=uint8  DataLength=1  NoAck=off  RepeatedStart=off  OutputStatus=off  blockPlatform=ARDUINO
  x 100 : Gain  Gain=100
  wires:
  command [mA]/1 -> x 100/1
  x 100/1 -> Data Type Conversion/1
  Data Type Conversion/1 -> I2C Write (0xB0)/1

== system roller485lib/Basic I2C Write/basic relative angle command [deg] ==
  command [deg] : Inport
  Clock : Clock
  Compare To Constant : simulink/Logic and Bit Operations/Compare To Constant  relop===  const=0  OutDataTypeStr=boolean
  Data Type Conversion : DataTypeConversion  OutDataTypeStr=uint32  SaturateOnIntegerOverflow=off  RndMeth=Floor
  Enabled Subsystem (initialization angle) : Subsystem  TreatAsAtomicUnit=on
  I2C Write (0x80) : arduinolib/I2C Write  I2CModule=0  Mode=Master  SlaveAddress=I2CAddress  SlaveByteOrder=LittleEndian  Direction=Transmitter  RegisterAddressMode=on  RegisterAddress=0x80  SlaveDataType=uint8  DataLength=1  NoAck=off  RepeatedStart=off  OutputStatus=off  blockPlatform=ARDUINO
  Sum : Sum  Inputs=++|
  x 100 : Gain  Gain=100
  wires:
  Compare To Constant/1 -> Enabled Subsystem (initialization angle)/Enable
  Clock/1 -> Compare To Constant/1
  command [deg]/1 -> Sum/2
  Enabled Subsystem (initialization angle)/1(initial angle) -> Sum/1
  Sum/1 -> x 100/1
  Data Type Conversion/1 -> I2C Write (0x80)/1
  x 100/1 -> Data Type Conversion/1

== system roller485lib/Basic I2C Write/basic relative angle command [rad] ==
  command [rad] : Inport
  Clock : Clock
  Compare To Constant : simulink/Logic and Bit Operations/Compare To Constant  relop===  const=0  OutDataTypeStr=boolean
  Data Type Conversion : DataTypeConversion  OutDataTypeStr=uint32  SaturateOnIntegerOverflow=off  RndMeth=Floor
  Enabled Subsystem (initialization angle) : Subsystem  TreatAsAtomicUnit=on
  I2C Write (0x80) : arduinolib/I2C Write  I2CModule=0  Mode=Master  SlaveAddress=I2CAddress  SlaveByteOrder=LittleEndian  Direction=Transmitter  RegisterAddressMode=on  RegisterAddress=0x80  SlaveDataType=uint8  DataLength=1  NoAck=off  RepeatedStart=off  OutputStatus=off  blockPlatform=ARDUINO
  Sum : Sum  Inputs=++|
  rad to deg : Gain  Gain=180/pi
  x 100 : Gain  Gain=100
  wires:
  Enabled Subsystem (initialization angle)/1(initial angle) -> Sum/1
  command [rad]/1 -> rad to deg/1
  Clock/1 -> Compare To Constant/1
  Compare To Constant/1 -> Enabled Subsystem (initialization angle)/Enable
  Data Type Conversion/1 -> I2C Write (0x80)/1
  x 100/1 -> Data Type Conversion/1
  Sum/1 -> x 100/1
  rad to deg/1 -> Sum/2

== system roller485lib/Basic I2C Write/position PID ==
  " x 10^5 " : Gain  Gain=1e5
  D : Constant  Value=position_D
  Data Type Conversion1 : DataTypeConversion  OutDataTypeStr=uint32  SaturateOnIntegerOverflow=off  RndMeth=Floor
  Data Type Conversion2 : DataTypeConversion  OutDataTypeStr=uint32  SaturateOnIntegerOverflow=off  RndMeth=Floor
  Data Type Conversion3 : DataTypeConversion  OutDataTypeStr=uint32  SaturateOnIntegerOverflow=off  RndMeth=Floor
  I : Constant  Value=position_I
  I2C Write (0xA0) : arduinolib/I2C Write  I2CModule=0  Mode=Master  SlaveAddress=I2CAddress  SlaveByteOrder=LittleEndian  Direction=Transmitter  RegisterAddressMode=on  RegisterAddress=0xA0  SlaveDataType=uint8  DataLength=1  NoAck=off  RepeatedStart=off  OutputStatus=off  blockPlatform=ARDUINO
  I2C Write (0xA4) : arduinolib/I2C Write  I2CModule=0  Mode=Master  SlaveAddress=I2CAddress  SlaveByteOrder=LittleEndian  Direction=Transmitter  RegisterAddressMode=on  RegisterAddress=0xA4  SlaveDataType=uint8  DataLength=1  NoAck=off  RepeatedStart=off  OutputStatus=off  blockPlatform=ARDUINO
  I2C Write (0xA8) : arduinolib/I2C Write  I2CModule=0  Mode=Master  SlaveAddress=I2CAddress  SlaveByteOrder=LittleEndian  Direction=Transmitter  RegisterAddressMode=on  RegisterAddress=0xA8  SlaveDataType=uint8  DataLength=1  NoAck=off  RepeatedStart=off  OutputStatus=off  blockPlatform=ARDUINO
  P : Constant  Value=position_P
  x 10^5 : Gain  Gain=1e5
  x 10^7 : Gain  Gain=1e7
  wires:
  P/1 -> x 10^5/1
  I/1 -> x 10^7/1
  D/1 -> " x 10^5 "/1
  Data Type Conversion1/1 -> I2C Write (0xA0)/1
  Data Type Conversion3/1 -> I2C Write (0xA8)/1
  Data Type Conversion2/1 -> I2C Write (0xA4)/1
  x 10^5/1 -> Data Type Conversion1/1
  x 10^7/1 -> Data Type Conversion2/1
  " x 10^5 "/1 -> Data Type Conversion3/1

== system roller485lib/Basic I2C Write/position PID (within set time) ==
  Clock : Clock
  Compare To Constant : simulink/Logic and Bit Operations/Compare To Constant  relop=<=  const=set_time  OutDataTypeStr=boolean
  D : Constant  Value=position_D
  Enabled Subsystem : Subsystem  TreatAsAtomicUnit=on
  I : Constant  Value=position_I
  P : Constant  Value=position_P
  wires:
  D/1 -> Enabled Subsystem/3(D)
  I/1 -> Enabled Subsystem/2(I)
  P/1 -> Enabled Subsystem/1(P)
  Compare To Constant/1 -> Enabled Subsystem/Enable
  Clock/1 -> Compare To Constant/1

== system roller485lib/Basic I2C Write/speed PID ==
  " x 10^5 " : Gain  Gain=1e5
  D : Constant  Value=speed_D
  Data Type Conversion2 : DataTypeConversion  OutDataTypeStr=uint32  SaturateOnIntegerOverflow=off  RndMeth=Floor
  Data Type Conversion4 : DataTypeConversion  OutDataTypeStr=uint32  SaturateOnIntegerOverflow=off  RndMeth=Floor
  Data Type Conversion6 : DataTypeConversion  OutDataTypeStr=uint32  SaturateOnIntegerOverflow=off  RndMeth=Floor
  I : Constant  Value=speed_I
  I2C Write (0x70) : arduinolib/I2C Write  I2CModule=0  Mode=Master  SlaveAddress=I2CAddress  SlaveByteOrder=LittleEndian  Direction=Transmitter  RegisterAddressMode=on  RegisterAddress=0x70  SlaveDataType=uint8  DataLength=1  NoAck=off  RepeatedStart=off  OutputStatus=off  blockPlatform=ARDUINO
  I2C Write (0x74) : arduinolib/I2C Write  I2CModule=0  Mode=Master  SlaveAddress=I2CAddress  SlaveByteOrder=LittleEndian  Direction=Transmitter  RegisterAddressMode=on  RegisterAddress=0x74  SlaveDataType=uint8  DataLength=1  NoAck=off  RepeatedStart=off  OutputStatus=off  blockPlatform=ARDUINO
  I2C Write (0x78) : arduinolib/I2C Write  I2CModule=0  Mode=Master  SlaveAddress=I2CAddress  SlaveByteOrder=LittleEndian  Direction=Transmitter  RegisterAddressMode=on  RegisterAddress=0x78  SlaveDataType=uint8  DataLength=1  NoAck=off  RepeatedStart=off  OutputStatus=off  blockPlatform=ARDUINO
  P : Constant  Value=speed_P
  x 10^5 : Gain  Gain=1e5
  x 10^7 : Gain  Gain=1e7
  wires:
  D/1 -> " x 10^5 "/1
  I/1 -> x 10^7/1
  P/1 -> x 10^5/1
  Data Type Conversion2/1 -> I2C Write (0x70)/1
  Data Type Conversion4/1 -> I2C Write (0x74)/1
  Data Type Conversion6/1 -> I2C Write (0x78)/1
  x 10^5/1 -> Data Type Conversion2/1
  x 10^7/1 -> Data Type Conversion4/1
  " x 10^5 "/1 -> Data Type Conversion6/1

== system roller485lib/Basic I2C Write/speed PID (within set time) ==
  Clock : Clock
  Compare To Constant : simulink/Logic and Bit Operations/Compare To Constant  relop=<=  const=set_time  OutDataTypeStr=boolean
  D : Constant  Value=speed_D
  Enabled Subsystem : Subsystem  TreatAsAtomicUnit=on
  I : Constant  Value=speed_I
  P : Constant  Value=speed_P
  wires:
  Clock/1 -> Compare To Constant/1
  Compare To Constant/1 -> Enabled Subsystem/Enable
  P/1 -> Enabled Subsystem/1(P)
  I/1 -> Enabled Subsystem/2(I)
  D/1 -> Enabled Subsystem/3(D)

== system roller485lib/Basic I2C Write (using MATLAB Function)/basic absolute angle command [deg] (using MATLAB Function) ==
  command [deg] : Inport
  I2C Write (0x80) : arduinolib/I2C Write  I2CModule=0  Mode=Master  SlaveAddress=I2CAddress  SlaveByteOrder=BigEndian  Direction=Transmitter  RegisterAddressMode=on  RegisterAddress=0x80  SlaveDataType=uint8  DataLength=1  NoAck=off  RepeatedStart=off  OutputStatus=off  blockPlatform=ARDUINO
  MATLAB Function : MATLAB Function  TreatAsAtomicUnit=on
  x 100 : Gain  Gain=100
  wires:
  command [deg]/1 -> x 100/1
  MATLAB Function/1(bytes) -> I2C Write (0x80)/1
  x 100/1 -> MATLAB Function/1(double_data)

== system roller485lib/Basic I2C Write (using MATLAB Function)/basic absolute angle command [rad] (using MATLAB Function) ==
  command [rad] : Inport
  I2C Write (0x80) : arduinolib/I2C Write  I2CModule=0  Mode=Master  SlaveAddress=I2CAddress  SlaveByteOrder=BigEndian  Direction=Transmitter  RegisterAddressMode=on  RegisterAddress=0x80  SlaveDataType=uint8  DataLength=1  NoAck=off  RepeatedStart=off  OutputStatus=off  blockPlatform=ARDUINO
  MATLAB Function : MATLAB Function  TreatAsAtomicUnit=on
  rad to deg : Gain  Gain=180/pi
  x 100 : Gain  Gain=100
  wires:
  x 100/1 -> MATLAB Function/1(double_data)
  MATLAB Function/1(bytes) -> I2C Write (0x80)/1
  command [rad]/1 -> rad to deg/1
  rad to deg/1 -> x 100/1

== system roller485lib/Basic I2C Write (using MATLAB Function)/basic angular velocity command [rad//s] (using MATLAB Function) ==
  command [rad/s] : Inport
  I2C Write (0x40) : arduinolib/I2C Write  I2CModule=0  Mode=Master  SlaveAddress=I2CAddress  SlaveByteOrder=BigEndian  Direction=Transmitter  RegisterAddressMode=on  RegisterAddress=0x40  SlaveDataType=uint8  DataLength=1  NoAck=off  RepeatedStart=off  OutputStatus=off  blockPlatform=ARDUINO
  MATLAB Function : MATLAB Function  TreatAsAtomicUnit=on
  rad/s to rpm : Gain  Gain=60/(2*pi)
  x 100 : Gain  Gain=100
  wires:
  MATLAB Function/1(bytes) -> I2C Write (0x40)/1
  command [rad/s]/1 -> rad/s to rpm/1
  rad/s to rpm/1 -> x 100/1
  x 100/1 -> MATLAB Function/1(double_data)
